simulink model "Test"  (R2022b)
settings: Solver=VariableStepAuto  StartTime=0.0  StopTime=inf  RelTol=1e-3
settings Model: Creator=sabat  LastModifiedBy=sabat

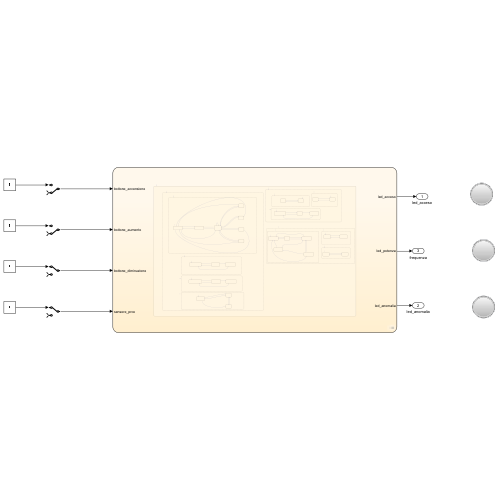
[thumbnail: Simulink's stored preview of the top-level diagram]
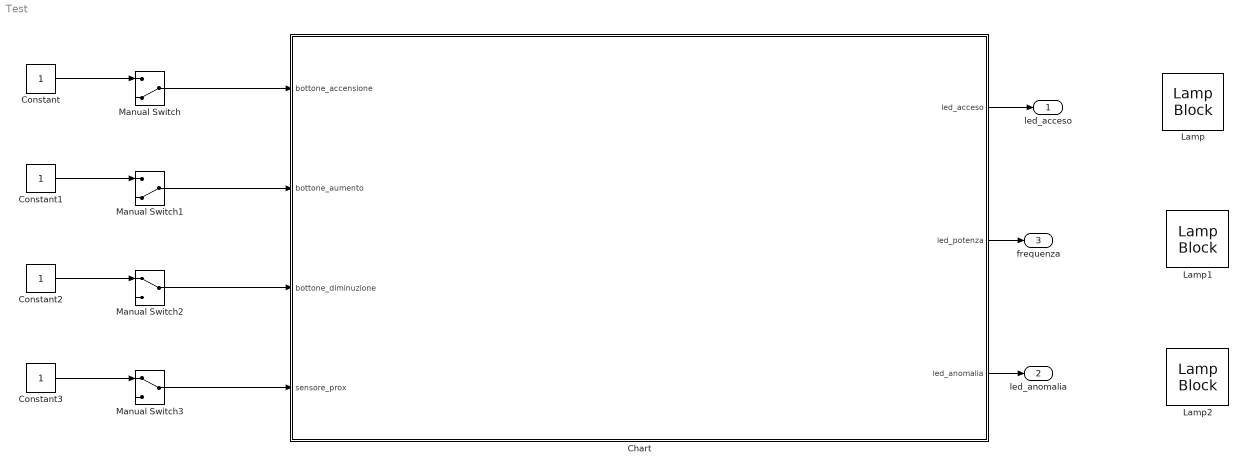
== system Test ==
  Chart : Stateflow chart  TreatAsAtomicUnit=on
  Constant{,1..3} (4 alike) : Constant
  Lamp : LampBlock  LabelPosition=Hide
  Lamp1 : LampBlock  LabelPosition=Hide
  Lamp2 : LampBlock  LabelPosition=Hide
  Manual Switch : ManualSwitch  CurrentSetting=0
  Manual Switch1 : ManualSwitch  CurrentSetting=0
  Manual Switch2 : ManualSwitch
  Manual Switch3 : ManualSwitch
  led_acceso : Outport
  led_anomalia : Outport  Port=2
  frequenza : Outport  Port=3
  wires:
  Manual Switch/1 -> Chart/1(bottone_accensione)
  Manual Switch1/1 -> Chart/2(bottone_aumento)
  Manual Switch2/1 -> Chart/3(bottone_diminuzione)
  Manual Switch3/1 -> Chart/4(sensore_prox)
  Constant/1 -> Manual Switch/1
  Constant1/1 -> Manual Switch1/1
  Constant2/1 -> Manual Switch2/1
  Constant3/1 -> Manual Switch3/1
  Chart/1(led_acceso) -> led_acceso/1
  Chart/3(led_anomalia) -> led_anomalia/1
  Chart/2(led_potenza) -> frequenza/1

== stateflow chart Test/Chart ==
  state Fornello_induzione
    state Accensione [parallel]
      settings: executionOrder=2
      state led_accensione [parallel]
        settings: executionOrder=3
        state led_acceso
          led_acceso=1;
        state led_spento
          led_acceso = 0;
        (default) -> Fornello_induzione.Accensione.led_accensione.led_spento
        Fornello_induzione.Accensione.led_accensione.led_acceso -> Fornello_induzione.Accensione.led_accensione.led_spento : [evento_spegnimento == 1]
        Fornello_induzione.Accensione.led_accensione.led_spento -> Fornello_induzione.Accensione.led_accensione.led_acceso : [bottone_accensione == 1 && evento_spegnimento == 0]
      state Logica_Accensione_Spegnimento [parallel]
        settings: executionOrder=1
        state Acceso
          acceso = 1;
        state Spento
          acceso = 0;
        (default) -> Spento
        Acceso -> Spento : [evento_spegnimento == 1]
        Spento -> Acceso : [bottone_accensione == 1 && evento_spegnimento == 0]
      state Bottone_Accensione [parallel]
        settings: executionOrder=2
        state NonPremuto
          evento_spegnimento = 0;
        state InPressione
        state Premuto
          evento_spegnimento = 1;
        (default) -> NonPremuto
        InPressione -> Premuto [order 2] : [after(1,sec)]
        NonPremuto -> InPressione : [bottone_accensione == 1 && acceso == 1]
        InPressione -> NonPremuto [order 1] : [bottone_accensione == 0]
        Premuto -> NonPremuto : [bottone_accensione == 0]
      (default) -> led_accensione [order 3]
      (default) -> Logica_Accensione_Spegnimento [order 1]
      (default) -> Bottone_Accensione [order 2]
    state Cambiamento_Potenza_Fornello [parallel]
      settings: executionOrder=1
      state Gestione_Potenza [parallel]
        settings: executionOrder=1
        state Potenza_300
          potenza=300;
          frequenza=2;
          attivo = 1;
        state Potenza_500
          potenza=500;
          frequenza=1;
          attivo = 1;
        state Appoggio
          en: app = contatore;
        state Potenza_Attivabile
          potenza = 0;
          attivo = 0;
          frequenza = 0;
        state Potenza_Non_Attivabile
          contatore = 0;
          potenza = 0;
          frequenza = 0;
        state Potenza_1000
          potenza=1000;
          frequenza=0.5;
          attivo = 1;
        state Potenza_1500
          potenza=1500;
          frequenza=0.25;
          attivo = 1;
        Potenza_500 -> Potenza_Non_Attivabile [order 2] : [disattivaFornello == 1 || acceso == 0]
        Potenza_300 -> Potenza_Non_Attivabile [order 2] : [disattivaFornello == 1 || acceso == 0]
        Appoggio -> Potenza_300 [order 2] : [after(5,sec) && contatore == 1]
        Potenza_300 -> Appoggio [order 1] : [contatore ~= 1]
        Appoggio -> Potenza_500 [order 4] : [after(5,sec) && contatore == 2]
        Potenza_500 -> Appoggio [order 1] : [contatore ~= 2]
        Appoggio -> Appoggio [order 3] : [app ~= contatore]
        (default) -> Potenza_Non_Attivabile
        Potenza_Non_Attivabile -> Potenza_Attivabile : [pentola == 1]
        Potenza_Attivabile -> Appoggio [order 2] : [contatore ~= 0]
        Potenza_Attivabile -> Potenza_Non_Attivabile [order 1] : [pentola == 0]
        Appoggio -> Potenza_Attivabile [order 1] : [after(5,sec) && contatore == 0]
        Appoggio -> Potenza_1000 [order 5] : [after(5,sec) && contatore == 3]
        Potenza_1000 -> Appoggio [order 1] : [contatore ~= 3]
        Potenza_1000 -> Potenza_Non_Attivabile [order 2] : [disattivaFornello == 1 || acceso == 0]
        Potenza_1500 -> Potenza_Non_Attivabile [order 2] : [disattivaFornello == 1 || acceso == 0]
        Appoggio -> Potenza_Non_Attivabile [order 7] : [disattivaFornello == 1 || acceso == 0 ]
        Potenza_1500 -> Appoggio [order 1] : [contatore ~= 4]
        Appoggio -> Potenza_1500 [order 6] : [after(5,sec) && contatore == 4]
      state Bottone_Aumento [parallel]
        settings: executionOrder=2
        state Non_Premuto_Aumento_Potenza
        state In_Pressione_Aumento
        state PremutoAumento
          en: contatore = contatore + 1;
        (default) -> Non_Premuto_Aumento_Potenza
        In_Pressione_Aumento -> PremutoAumento [order 2] : [after(1,sec)]
        Non_Premuto_Aumento_Potenza -> In_Pressione_Aumento : [bottone_aumento == 1 && bottone_diminuzione == 0]
        In_Pressione_Aumento -> Non_Premuto_Aumento_Potenza [order 1] : [bottone_aumento == 0 || contatore == 4 || acceso == 0]
        PremutoAumento -> Non_Premuto_Aumento_Potenza : [bottone_aumento == 0 || acceso == 0]
      state Bottone_Diminuzione [parallel]
        settings: executionOrder=3
        state Non_Premuto_Diminuzione_Potenza
        state In_Pressione_Dimuzione
        state Premuto_Diminuzione
          en: contatore = contatore - 1;
        (default) -> Non_Premuto_Diminuzione_Potenza
        In_Pressione_Dimuzione -> Premuto_Diminuzione [order 2] : [after(1,sec)]
        Non_Premuto_Diminuzione_Potenza -> In_Pressione_Dimuzione : [bottone_diminuzione == 1 && bottone_aumento == 0]
        In_Pressione_Dimuzione -> Non_Premuto_Diminuzione_Potenza [order 1] : [bottone_diminuzione == 0 || contatore == 0 || acceso == 0]
        Premuto_Diminuzione -> Non_Premuto_Diminuzione_Potenza : [bottone_diminuzione == 0 || acceso == 0]
      state Toggling_Led [parallel]
        settings: executionOrder=4
        state led_spento
          led_potenza = 0;
        state Led_Non_Attivabile
          led_potenza = 0;
        state led_acceso
          led_potenza = 1;
        Led_Non_Attivabile -> Fornello_induzione.Cambiamento_Potenza_Fornello.Toggling_Led.led_spento : [acceso == 1 && frequenza ~= 0 ]
        (default) -> Led_Non_Attivabile
        Fornello_induzione.Cambiamento_Potenza_Fornello.Toggling_Led.led_spento -> Led_Non_Attivabile [order 2] : [acceso == 0 || disattivaFornello == 1 || frequenza ==0 ]
        Fornello_induzione.Cambiamento_Potenza_Fornello.Toggling_Led.led_spento -> Fornello_induzione.Cambiamento_Potenza_Fornello.Toggling_Led.led_acceso [order 1] : [after(frequenza,sec) && frequenza ~= 0]
        Fornello_induzione.Cambiamento_Potenza_Fornello.Toggling_Led.led_acceso -> Fornello_induzione.Cambiamento_Potenza_Fornello.Toggling_Led.led_spento [order 1] : [after(frequenza, sec) && frequenza ~= 0]
        Fornello_induzione.Cambiamento_Potenza_Fornello.Toggling_Led.led_acceso -> Led_Non_Attivabile [order 2] : [acceso == 0 || disattivaFornello == 1 || frequenza == 0]
      (default) -> Gestione_Potenza [order 4]
      (default) -> Bottone_Aumento [order 1]
      (default) -> Bottone_Diminuzione [order 2]
      (default) -> Toggling_Led [order 3]
    state Prossimita_Pentola [parallel]
      settings: executionOrder=3
      state Logica_Sensore_Pentola [parallel]
        settings: executionOrder=1
        state SensoreNonAttivato
          disattivaFornello = 0;
          accendi_led_anomalia = 0;
          pentola = 0;
        state SensoreAttivato
          anomalia = 0;
        state RilevamentoPentola
          accendi_led_anomalia = 0;
          disattivaFornello = 0;
        state DisattivaFornello
          disattivaFornello = 1;
          accendi_led_anomalia = 0;
          pentola = 0;
        state Allarme
          accendi_led_anomalia = 1;
        RilevamentoPentola -> SensoreNonAttivato [order 3] : [acceso == 0]
        (default) -> SensoreNonAttivato
        SensoreAttivato -> RilevamentoPentola [order 2] : [pentola == 1]
        SensoreNonAttivato -> SensoreAttivato : [acceso == 1]
        SensoreAttivato -> SensoreNonAttivato [order 1] : [acceso == 0]
        RilevamentoPentola -> SensoreAttivato [order 1] : [pentola == 0 && attivo == 0]
        Allarme -> SensoreNonAttivato [order 2] : [acceso == 0]
        DisattivaFornello -> SensoreNonAttivato [order 2] : [acceso == 0]
        DisattivaFornello -> RilevamentoPentola [order 1] : [pentola == 1]
        Allarme -> RilevamentoPentola [order 1] : [pentola == 1]
        RilevamentoPentola -> Allarme [order 2] : [pentola == 0 && attivo == 1]
        Allarme -> DisattivaFornello [order 3] : [after(10,sec) && pentola == 0]
      state Sensore_Prossimita [parallel]
        settings: executionOrder=2
        state Pentola_assente
          pentola = 0;
        state Pentola_Presente
          pentola = 1;
        (default) -> Pentola_assente
        Pentola_assente -> Pentola_Presente : [sensore_prox == 1 && acceso == 1]
        Pentola_Presente -> Pentola_assente : [sensore_prox == 0 || acceso == 0]
      state Led_Anomalia [parallel]
        settings: executionOrder=3
        state Led_spento
          led_anomalia = 0;
        state Led_Acceso
          led_anomalia = 1;
        (default) -> Led_spento
        Led_spento -> Led_Acceso : [accendi_led_anomalia == 1]
        Led_Acceso -> Led_spento : [accendi_led_anomalia == 0]
      (default) -> Logica_Sensore_Pentola [order 1]
      (default) -> Sensore_Prossimita [order 2]
      (default) -> Led_Anomalia [order 3]
    (default) -> Accensione [order 1]
    (default) -> Cambiamento_Potenza_Fornello [order 3]
    (default) -> Prossimita_Pentola [order 2]
  (default) -> Fornello_induzione
  data: bottone_accensione input; bottone_aumento input; bottone_diminuzione input; sensore_prox input; acceso local; app local; attivo local; contatore local; disattivaFornello local; evento_spegnimento local; pentola local; anomalia local; led_acceso output; potenza local; led_potenza output; frequenza local =0; accendi_led_anomalia local; led_anomalia output
